simulink model "FULLWAVEwithR"  (Simulink 7.5)
settings: Solver=ode45  StartTime=0.0  StopTime=1  RelTol=1e-3
undefined symbols (not defined in the file): deg
libraries: powerlib x9, powerlib_extras x4
settings Model: Creator=Singhal  LastModifiedBy=Singhal

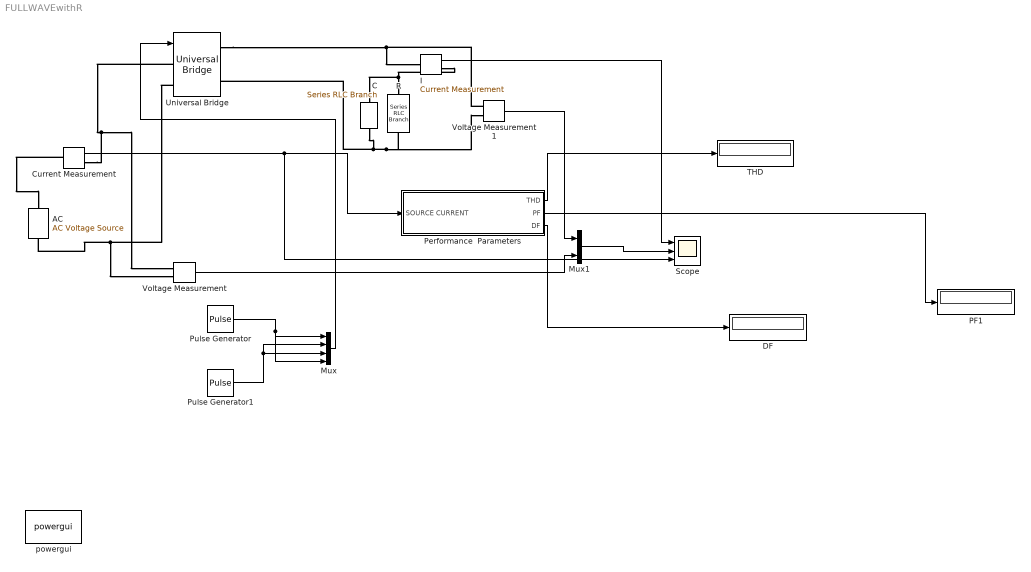
== system FULLWAVEwithR ==
  "AC " : powerlib/Electrical Sources/AC Voltage Source  DialogController=POWERSYS.PowerSysDialog  SystemSampleTime=-1  Amplitude=100  Phase=0  Frequency=50  SampleTime=0  Measurements=None
  C : powerlib/Elements/Series RLC Branch  DialogController=POWERSYS.PowerSysDialog  PhysicalDomain=powersysdomain  SubClassName=unknown  LeftPortType=p1  RightPortType=p1  LConnTagsString=__new0  RConnTagsString=__new0  BranchType=C  Resistance=10  Inductance=0.1  SetiL0=off  InitialCurrent=0  Capacitance=1e-6  Setx0=off  InitialVoltage=0  Measurements=None
  Current Measurement : powerlib/Measurements/Current Measurement  DialogController=POWERSYS.PowerSysDialog  SystemSampleTime=-1  PhasorSimulation=off  OutputType=Complex  PSBequivalent=0
  DF : Display
  I : powerlib/Measurements/Current Measurement  DialogController=POWERSYS.PowerSysDialog  SystemSampleTime=-1  PhasorSimulation=off  OutputType=Complex  PSBequivalent=0
  Mux : Mux
  Mux1 : Mux  Inputs=2
  PF1 : Display
  Performance  Parameters : Subsystem
  Pulse Generator : DiscretePulseGenerator  PulseType=Time based  Amplitude=1  Period=0.02  PulseWidth=5  PhaseDelay=deg/18000  SampleTime=1
  Pulse Generator1 : DiscretePulseGenerator  PulseType=Time based  Amplitude=1  Period=0.02  PulseWidth=5  PhaseDelay=(deg+180)/18000  SampleTime=1
  R : powerlib/Elements/Series RLC Branch  DialogController=POWERSYS.PowerSysDialog  PhysicalDomain=powersysdomain  SubClassName=unknown  LeftPortType=p1  RightPortType=p1  LConnTagsString=__new0  RConnTagsString=__new0  BranchType=R  Resistance=10  Inductance=0.1  SetiL0=off  InitialCurrent=0  Capacitance=1e-6  Setx0=off  InitialVoltage=0  Measurements=None
  Scope : Scope  NumInputPorts=3
      settings: TimeRange=0.25  YMin=-100~-5~-5  YMax=100~5~5
  THD : Display
  Universal Bridge : powerlib/Power Electronics/Universal Bridge  DialogController=POWERSYS.PowerSysDialog  SystemSampleTime=-1  Arms=2  SnubberResistance=1e5  SnubberCapacitance=inf  Device=Thyristors  Ron=1e-3  Lon=0  ForwardVoltages="[  0  0  ]"  ForwardVoltage=0  GTOparameters=[ 10e-6 , 20e-6 ]  IGBTparameters=[ 1e-6 , 2e-6 ]  Measurements=None  Measurements_2=None  converterType=Rectifier
  Voltage Measurement : powerlib/Measurements/Voltage Measurement  DialogController=POWERSYS.PowerSysDialog  SystemSampleTime=-1  PhasorSimulation=off  OutputType=Complex  PSBequivalent=0
  Voltage Measurement1 : powerlib/Measurements/Voltage Measurement  DialogController=POWERSYS.PowerSysDialog  SystemSampleTime=-1  PhasorSimulation=off  OutputType=Complex  PSBequivalent=0
  powergui : powerlib/powergui  Priority=1  SystemSampleTime=-1  SimulationMode=Discrete  SampleTime=50e-6  frequency=60  SPID=off  DisableSnubberDevices=off  DisableRonSwitches=off  DisableVfSwitches=off  SwTol=0  Interpol=off  frequencyindice=50  echomessages=off  HookPort=off  DisplayEquations=off  FunctionMessages=off  EnableUseOfTLC=off  x0status=blocks  RestoreLinks=warning  ResistiveCurrentMeasurement=off  Ylog=off  Xlog=on  ShowGrid=off  save=off  variable=ZData  ZoomFFT=off  StartTime=0.0  cycles=1  DisplayStyle=1  FreqAxis=off  MaxFrequency=1000  frequencyindicesteady=1  display=off  methode=off
  wires:
  Pulse Generator/1 -> Mux/1, Mux/4
  Pulse Generator1/1 -> Mux/2, Mux/3
  Mux/1 -> Universal Bridge/1
  Voltage Measurement/1 -> Mux1/2
  Voltage Measurement1/1 -> Mux1/1
  Performance  Parameters/1(THD) -> THD/1
  Performance  Parameters/3(DF) -> DF/1
  Performance  Parameters/2(PF) -> PF1/1
  Current Measurement/1 -> Performance  Parameters/1(SOURCE CURRENT), Scope/3
  Mux1/1 -> Scope/2
  I/1 -> Scope/1
  connections:
  Universal Bridge/LConn1 -- Voltage Measurement/LConn1 -- Current Measurement/RConn1
  "AC "/LConn1 -- Voltage Measurement/LConn2 -- Universal Bridge/LConn2
  Universal Bridge/RConn1 -- Voltage Measurement1/LConn1 -- I/LConn1
  Voltage Measurement1/LConn2 -- R/RConn1 -- Universal Bridge/RConn2 -- C/RConn1
  Current Measurement/LConn1 -- "AC "/RConn1
  I/RConn1 -- R/LConn1 -- C/LConn1

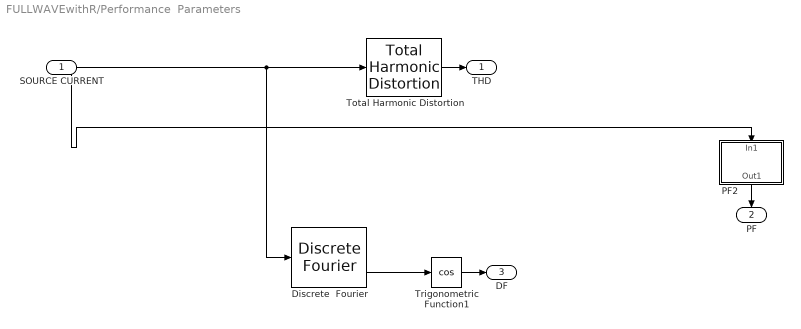
== system FULLWAVEwithR/Performance  Parameters ==
  SOURCE CURRENT : Inport
  Discrete  Fourier : powerlib_extras/Discrete Measurements/Discrete  Fourier  DialogController=POWERSYS.PowerSysDialog  SystemSampleTime=-1  Freq=50  n=1  Par_Init=[0 0]  Ts=50e-6
  PF2 : Subsystem
  Total Harmonic Distortion : powerlib_extras/Measurements/Total Harmonic Distortion  DialogController=POWERSYS.PowerSysDialog  SystemSampleTime=-1  f1=50
  Trigonometric Function1 : Trigonometry  Operator=cos
  THD : Outport
  PF : Outport  Port=2
  DF : Outport  Port=3
  wires:
  SOURCE CURRENT/1 -> PF2/1(In1), Discrete  Fourier/1, Total Harmonic Distortion/1
  Discrete  Fourier/2 -> Trigonometric Function1/1
  Total Harmonic Distortion/1 -> THD/1
  PF2/1(Out1) -> PF/1
  Trigonometric Function1/1 -> DF/1

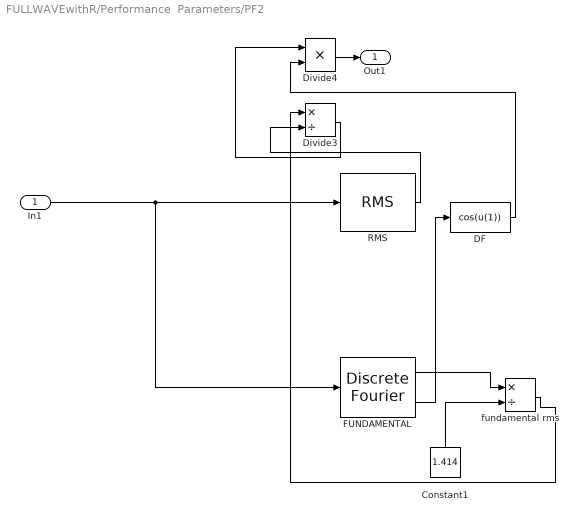
== system FULLWAVEwithR/Performance  Parameters/PF2 ==
  In1 : Inport
  Constant1 : Constant  Value=1.414  OutDataType=fixdt(1, 16)  OutScaling=2^0
  DF : Fcn  Expr=cos(u(1))
  Divide3 : Product  Inputs=*/  OutDataType=fixdt(1, 16)  OutScaling=2^-10
  Divide4 : Product  Inputs=**  OutDataType=fixdt(1, 16)  OutScaling=2^-10
  FUNDAMENTAL : powerlib_extras/Discrete Measurements/Discrete  Fourier  DialogController=POWERSYS.PowerSysDialog  SystemSampleTime=-1  Freq=50  n=1  Par_Init=[0 0]  Ts=50e-3
  RMS : powerlib_extras/Measurements/RMS  DialogController=POWERSYS.PowerSysDialog  SystemSampleTime=-1  f1=50
  fundamental rms : Product  Inputs=*/  OutDataType=fixdt(1, 16)  OutScaling=2^-10
  Out1 : Outport
  wires:
  DF/1 -> Divide4/2
  Divide3/1 -> Divide4/1
  fundamental rms/1 -> Divide3/1
  FUNDAMENTAL/1 -> fundamental rms/1
  FUNDAMENTAL/2 -> DF/1
  Constant1/1 -> fundamental rms/2
  Divide4/1 -> Out1/1
  In1/1 -> RMS/1, FUNDAMENTAL/1
  RMS/1 -> Divide3/2
